simulink model "chap6_6sim"  (Simulink 7.7)
settings: Solver=ode23  StartTime=0.0  StopTime=20  RelTol=1e-3
settings Model: Creator=yrx  LastModifiedBy=ljk
settings DataIOCC: SignalLoggingName=sigsOut
settings OptimizationCC: InitFltsAndDblsToZero=on
settings DebuggingCC: SaveWithParameterizedLinksMsg=none  SignalResolutionControl=TryResolveAllWithWarning  SolverPrmCheckMsg=none  MultiTaskDSMMsg=warning  MultiTaskCondExecSysMsg=none  StrictBusMsg=None
settings HardwareCC: TargetUnknown=on
settings RTWCC: IncludeERTFirstTime=on

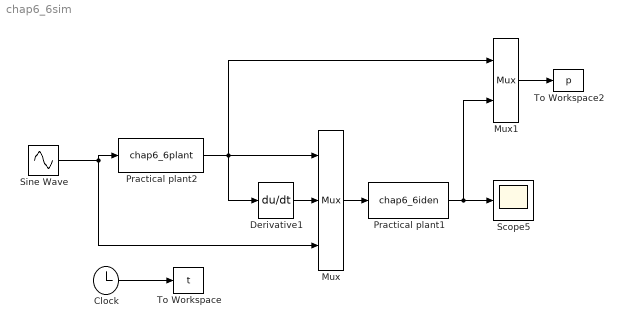
== system chap6_6sim ==
  Clock : Clock
      settings: Decimation=10
  Derivative1 : Derivative
  Mux : Mux  Inputs=3
  Mux1 : Mux  Inputs=2
  Practical plant1 : S-Function  FunctionName=chap6_6iden  EnableBusSupport=off
  Practical plant2 : S-Function  FunctionName=chap6_6plant  EnableBusSupport=off
  Scope5 : Scope
      settings: YMin=-30  YMax=140  SaveName=ScopeData5  MaxDataPoints=50000
  Sine Wave : Sin  Amplitude=0.50  Frequency=30*pi  SampleTime=0
  To Workspace : ToWorkspace  VariableName=t  SampleTime=-1  SaveFormat=Array
  To Workspace2 : ToWorkspace  VariableName=p  SampleTime=-1  SaveFormat=Array
  wires:
  Mux/1 -> Practical plant1/1
  Practical plant1/1 -> Scope5/1, Mux1/2
  Practical plant2/1 -> Mux/1, Derivative1/1, Mux1/1
  Sine Wave/1 -> Practical plant2/1, Mux/3
  Derivative1/1 -> Mux/2
  Clock/1 -> To Workspace/1
  Mux1/1 -> To Workspace2/1
